simulink model "sm_car_4post_testrig"  (R2021b)
settings: Solver=ode23t  StartTime=0.0  StopTime=20  MaxStep=0.4  RelTol=1e-3  AbsTol=1e-3  EnableMultiTasking=on
PreLoadFcn:
  | sm_car_4post_param
  | sm_car_4post_param_posts
  | load sm_car_4post_op_01
  | load sm_car_4post_op_02
  | load sm_car_4post_op_03
  | 
  | 
  | sm_car_4post_vehicle_01_data
  | sm_car_4post_vehicle_02_data
  | sm_car_4post_vehicle_03_data
  | sm_car_4post_init_data
  | Vehicle = Vehicle_01;
  | sm_car_4post_op = sm_car_4post_op_01;
values from neighbouring files (symbols this model uses):
  brake_pressure_factor = 0.1    [sm_car_4post_param.m]
  brake_rear_factor = 0.3    [sm_car_4post_param.m]
  Init = struct    [sm_car_4post_init_data.m]
  N = 100    [sm_extr_data_cam_roller_curve.m]
  s = sin(q)    [sm_extr_data_cam_roller_curve.m]
  sm_car_4post_op_01 = simscape.op.create(simlog_sm_car_4post,20)    [sm_car_4post_gen_op.m]
  Vehicle_01 = struct    [sm_car_4post_vehicle_01_data.m]
undefined symbols (not defined in the file or in its folder): Axle, Hub, ShaftF, ShaftR, smcar_param, X, xy_data_car_side, xy_data_membrane, Y, Z
libraries: fl_lib x68, sm_lib x50, nesl_utility x40, sm_car_4post_lib x34, simulink x2
(part 1 of 4)
CloseFcn:
  | try,close(h1_sm_car_4post_testrig),end
  | clear h1_sm_car_4post_testrig
  | try,close(h2_sm_car_4post_testrig),end
  | clear h2_sm_car_4post_testrig
  | 
  | clear simlog_sm_car_4post_testrig
  | clear logsout_sm_car_4post_testrig
  | 
  | clear Init
  | clear Vehicle
  | clear Vehicle_01
  | clear Vehicle_02
  | clear Vehicle_03
  | clear brake_pressure_factor
  | clear brake_rear_factor
  | clear sm_car_4post_color
  | clear sm_car_4post_density
  | clear sm_car_4post_op
  | clear sm_car_4post_op_01
  | clear sm_car_4post_op_02
  | clear sm_car_4post_op_03
  | clear sm_car_4post_platform
  | clear smcar_param
  | clear xy_data_membrane
Description:
  | Full Vehicle on Four Post Testrig
settings Model: Creator=The MathWorks, Inc.  LastModifiedBy=The MathWorks, Inc.
settings SolverCC: ConcurrentTasks=on  AlgebraicLoopSolver=TrustRegion  AutoInsertRateTranBlk=on  InsertRTBMode=Never (minimum delay)
settings DataIOCC: MaxDataPoints=10000  SaveFormat=StructureWithTime  ReturnWorkspaceOutputs=off  SignalLoggingName=logsout_sm_car_4post_testrig
settings OptimizationCC: BlockReduction=off  OptimizeBlockIOStorage=off  BufferReuse=off  GlobalBufferReuse=off  ExpressionFolding=off  LocalBlockOutputs=off  OptimizeDataStoreBuffers=off  BusAssignmentInplaceUpdate=off
settings DebuggingCC: SFMachineParentedDataDiag=warning  ArithmeticOperatorsInVariantConditions=warning
settings HardwareCC: ProdBitPerPointer=32  ProdBitPerSizeT=32  ProdBitPerPtrDiffT=32  ProdLargestAtomicFloat=None  ProdWordSize=32  ProdLongLongMode=on  ProdHWDeviceType=Generic->32-bit x86 compatible
settings SFSimCC: CustomCodeUndefinedFunction=UseInterfaceOnly
settings RTWCC: RTWCompilerOptimization=on
settings GRTTargetCC: TargetLangStandard=C89/C90 (ANSI)
settings SimscapeCC: SimscapeLogType=all  SimscapeLogSimulationStatistics=on  SimscapeLogName=simlog_sm_car_4post_testrig  SimscapeLogDataHistory=100000  SimscapeUseOperatingPoints=on  SimscapeOperatingPoint=sm_car_4post_op
settings DiagnosticsConfigSet: SimMechanicsConflictingReferenceFrames=none  SimMechanicsRigidlyBoundBlock=none  SimMechanicsUnsatisfiedHighPriorityTargets=error
settings ExplorerConfigSet: InternalSimMechanicsExplorerSettings="<ExplorerConfiguration><canonicalview>default</canonicalview><AnimationSetting><BasePlaybackSpeed>1.0</BasePlaybackSpeed><PlaybackSpeedFactor>2.0</PlaybackSpeedFactor></AnimationSetting><TilePanel><TileInfo><Tiles Columns=\"2\" Count=\"3\" Rows=\"2\"><Column Weight=\"0.4993\"/><Column Weight=\"0.5007\"/><Row Weight=\"0.5\"/><Row Weight=\"0.5\"/><Tile Height=\"1\" Width=\"1\" X=\"0\" Y=\"0\"/><Tile Height=\"1\" Width=\"1\" X=\"1\" Y=\"0\"/><Tile Height=\"1\" Width=\"2\" X=\"0\" Y=\"1\"/></Tiles></TileInfo><SceneInfo><SceneViewer><BGColor><R>1</R><G>1</G><B>1</B></BGColor><Camera><DoPerspective>off</DoPerspective><Position><X>-193.503182231100908</X><Y>-61.0419033263629984</Y><Z>200.880247292376964</Z></Position><Center><X>-0.0764520266245204833</X><Y>0.688462788949241178</Y><Z>0.441979080031284555</Z></Center><Up><X>0.696897777137974517</X><Y>0.114900599241424928</Y><Z>0.707906307723070949</Z></Up><ViewLimDist>1</ViewLimDist><YLim>0.497951895852590032</YLim><XLim>0.688180709998523321</XLim></Camera></SceneViewer><SceneViewer><BGColor><R>1</R><G>1</G><B>1</B></BGColor><Camera><DoPerspective>off</DoPerspective><Position><X>-1.81478949286671787</X><Y>-285.659072572391551</Y><Z>0.350812117947062074</Z></Position><Center><X>-1.81478949286671787</X><Y>1.0996689468301124e-05</Y><Z>0.350812117947062074</Z></Center><Up><X>0</X><Y>-0</Y><Z>1</Z></Up><ViewLimDist>1</ViewLimDist><YLim>1.90555005908736064</YLim><XLim>2.64064989461544375</XLim></Camera></SceneViewer><SceneViewer><BGColor><R>1</R><G>1</G><B>1</B></BGColor><Camera><DoPerspective>off</DoPerspective><Position><X>174.747144460498959</X><Y>-221.722739064773151</Y><Z>43.636736806567896</Z></Position><Center><X>-1.89730184608775931</X><Y>-0.0435832957411751917</Y><Z>0.499781838173366855</Z></Center><Up><X>-0.0708368498921288503</X><Y>0.13584833277642594</Y><Z>0.988193994709149037</Z></Up><ViewLimDist>1</ViewLimDist><YLim>1.31510781083851214</YLim><XLim>3.68427206931538276</XLim></Camera></SceneViewer></SceneInfo></TilePanel><MechEditorPanel><Cameras><Camera><Id>Camera1</Id><Value><Name>Track Vehicle IsoRF</Name><NativeCamera><PositionTrackingFeature>Camera_Frames.Transform_Camera_BodyIso.F</PositionTrackingFeature><CenterTrackingFeature>Camera_Frames.Transform_Camera_BodyIso_Aim.F</CenterTrackingFeature><UpVectorTrackingFeature>Camera_Frames.Transform_Camera_BodyIso_Aim.F</UpVectorTrackingFeature><CenterTrackingOrigin>off</CenterTrackingOrigin><CenterTrackingDirection>+Y</CenterTrackingDirection><UpVectorTrackingDirection>+Z</UpVectorTrackingDirection></NativeCamera></Value></Camera><Camera><Id>Camera2</Id><Value><Name>Track Vehicle Rear</Name><NativeCamera><PositionTrackingFeature>Camera_Frames.Transform_Camera_Rear.F</PositionTrackingFeature><CenterTrackingFeature>Camera_Frames.Transform_Camera_Rear.F</CenterTrackingFeature><UpVectorTrackingFeature>Camera_Frames.World_Frame.W</UpVectorTrackingFeature><CenterTrackingOrigin>off</CenterTrackingOrigin><CenterTrackingDirection>+X</CenterTrackingDirection><UpVectorTrackingDirection>+Z</UpVectorTrackingDirection></NativeCamera></Value></Camera><Camera><Id>Camera3</Id><Value><Name>Track Vehicle Top</Name><NativeCamera><PositionTrackingFeature>Camera_Frames.Transform_Camera_Top.F</PositionTrackingFeature><CenterTrackingFeature>Camera_Frames.Transform_Camera_Top.F</CenterTrackingFeature><UpVectorTrackingFeature>Camera_Frames.Transform_Camera_Top.F</UpVectorTrackingFeature><CenterTrackingOrigin>off</CenterTrackingOrigin><CenterTrackingDirection>-Z</CenterTrackingDirection><UpVectorTrackingDirection>+X</UpVectorTrackingDirection></NativeCamera></Value></Camera><Camera><Id>Camera4</Id><Value><Name>Track Vehicle Right</Name><NativeCamera><PositionTrackingFeature>Camera_Frames.Transform_Camera_Right.F</PositionTrackingFeature><CenterTrackingFeature>Camera_Frames.Transform_Camera_Right.F</CenterTrackingFeature><UpVectorTrackingFeature>Camera_Frames.World_Frame.W</UpVectorTrackingFeature><CenterTrackingOrigin>off</CenterTrackingOrigin><CenterTrackingDirection>+Y</CenterTrackingDirection><UpVectorTrackingDirection>+Z</UpVectorTrackingDirection></NativeCamera></Value></Camera><Camera><Id>Camera5</Id><Value><Name>Track Susp FR</Name><NativeCamera><PositionTrackingFeature>Camera_Frames.Transform_Camera_Susp_FR.F</PositionTrackingFeature><CenterTrackingFeature>Camera_Frames.Transform_Camera_Susp_FR.F</CenterTrackingFeature><UpVectorTrackingFeature>Camera_Frames.World_Frame.W</UpVectorTrackingFeature><CenterTrackingOrigin>off</CenterTrackingOrigin><CenterTrackingDirection>-X</CenterTrackingDirection><UpVectorTrackingDirection>+Z</UpVectorTrackingDirection></NativeCamera></Value></Camera><Camera><Id>Camera6</Id><Value><Name>Track Susp RR</Name><NativeCamera><PositionTrackingFeature>Camera_Frames.Transform_Camera_Susp_RR.F</PositionTrackingFeature><CenterTrackingFeature>Camera_Frames.Transform_Camera_Susp_RR.F</CenterTrackingFeature><UpVectorTrackingFeature>Camera_Frames.Transform_Camera_Susp_RR.F</UpVectorTrackingFeature><CenterTrackingOrigin>off</CenterTrackingOrigin><CenterTrackingDirection>-X</CenterTrackingDirection><UpVectorTrackingDirection>+Z</UpVectorTrackingDirection></NativeCamera></Value></Camera></Cameras><GfxPanelCameraMap/><VideoCreator><PlaybackSpeedRatio>1.0</PlaybackSpeedRatio><FrameRate>30</FrameRate><VideoFormat>Motion JPEG AVI</VideoFormat><FrameSize>auto</FrameSize></VideoCreator></MechEditorPanel></ExplorerConfiguration>"

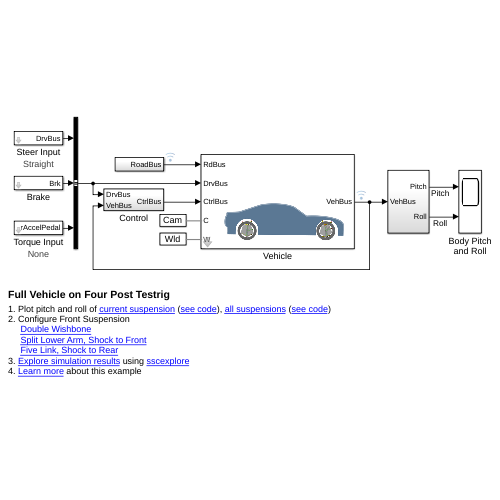
[thumbnail: Simulink's stored preview of the top-level diagram]
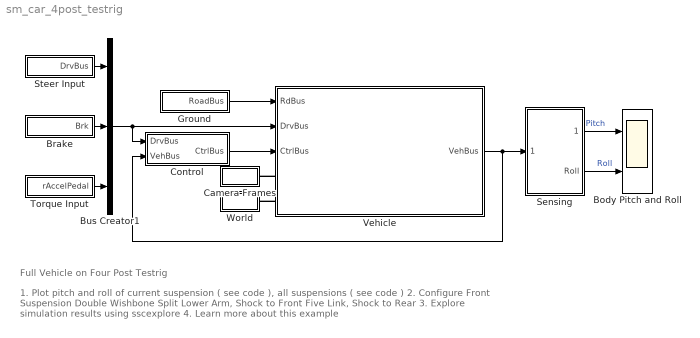
== system sm_car_4post_testrig ==
  note: Full Vehicle on Four Post Testrig
  note: 1. Plot pitch and roll of current suspension ( see code ), all suspensions ( see code )
      | 2. Configure Front Suspension
      | Double Wishbone
      | Split Lower Arm, Shock to Front
      | Five Link, Shock to Rear
      | 3. Explore simulation results using sscexplore
      | 4. Learn more about this example
  Body Pitch and Roll : Scope  NumInputPorts=2
  Brake : Subsystem  mask{brake_on_time=3600}
      mask prompts: brake_on_time "Brake On Time (sec)"
      mask TypeOptions brake_on_time: Step/Time
  Bus Creator1 : BusCreator  Inputs=3
  Camera Frames : Subsystem
      mask Display: disp('Cam')
  Control : Subsystem
  Ground : Subsystem
  Sensing : Subsystem
  Steer Input : Subsystem  mask{popup_steer_input=Straight}
      mask prompts: popup_steer_input "Steer Input"
      settings: AttributesFormatString=%<popup_steer_input>
      mask TypeOptions popup_steer_input: Straight | Step | Sequence | Lane Change
  Torque Input : Subsystem  mask{popup_torque_input=None}
      mask prompts: popup_torque_input "Maneuver Torque"
      mask init:
      | if (popup_torque_input == 1)
      |     rPedalValue = 0.5;
      | elseif (popup_torque_input == 2)
      |     rPedalValue = 0.25;
      | elseif (popup_torque_input == 3)
      |     rPedalValue = 0;
      | end
      settings: AttributesFormatString=%<popup_torque_input>
      mask TypeOptions popup_torque_input: Full Torque | Low Torque | None
  Vehicle : Subsystem  Tag=PublishSubsystem  VariantControl=NS_Con  mask(Vehicle with Multibody Suspension){Vehicle=Vehicle, Init=Init, InitTriggerDropdown=1}
      mask prompts: Vehicle "Vehicle Parameters"; Init "Initial Values"; InitTriggerDropdown "Initialization Trigger Dropdown"
      mask help: Multibody model of a car. All parameter values and the selected suspension configuration are defined by Vehicle Parameters, which must be a specific MATLAB data structure.
      mask init:
      | curblk = gcb;
      | 
      | % Trigger Mask Initialization for 
      | % variant subsystems below this level
      | sm_car_4post_lib_maskInitTrigger(curblk)
      mask TypeOptions InitTriggerDropdown: 0 | 1
      mask DialogControl cont_sim Prompt: Config
      mask Display: image(fullfile(matlabroot,'toolbox','physmod','sm','smdemos','car_4post_testrig','images','sm_car_4post_vehicle_sedan_IMAGE.png'));
  World : Subsystem
      mask Display: disp('Wld')
  wires:
  Bus Creator1/1 -> Control/1(DrvBus), Vehicle/2(DrvBus)
  Steer Input/1(DrvBus) -> Bus Creator1/1
  Brake/1(Brk) -> Bus Creator1/2
  Ground/1(RoadBus) -> Vehicle/1(RdBus)
  Torque Input/1(rAccelPedal) -> Bus Creator1/3
  Control/1(CtrlBus) -> Vehicle/3(CtrlBus)
  Vehicle/1(VehBus) -> Sensing/1(VehBus), Control/2(VehBus)
  Sensing/2(Roll) -> Body Pitch and Roll/2  "Roll"
  Sensing/1(Pitch) -> Body Pitch and Roll/1  "Pitch"
  connections:
  Vehicle/LConn2 -- World/RConn1
  Vehicle/LConn1 -- Camera Frames/RConn1

== system sm_car_4post_testrig/Brake ==
  Step : Step  Time=brake_on_time  After=0.5  SampleTime=0  ZeroCross=off
  Brk : Outport  VectorParamsAs1DForOutWhenUnconnected=off
  wires:
  Step/1 -> Brk/1  "rBrakePedal"

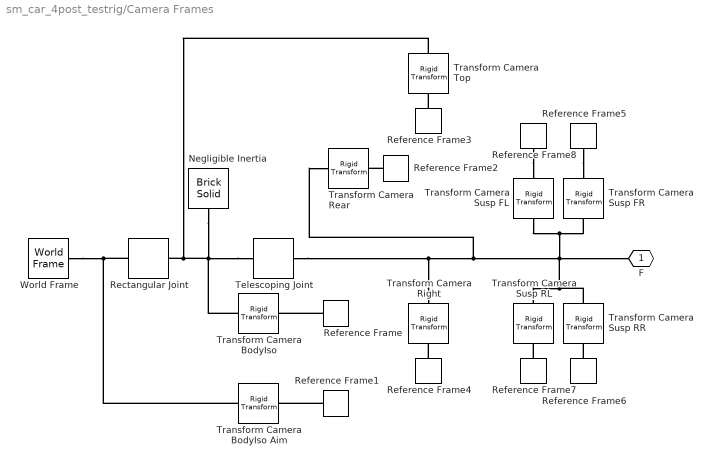
== system sm_car_4post_testrig/Camera Frames ==
  Negligible Inertia : sm_lib/Body Elements/Brick Solid  GraphicAmbientColor=[0.15 0.15 0.15 1.0]  BasedOnType=Density  BrickDimensions=[1 1 1]*1e-3  BrickDimensionUnits=m  CenterOfMass=[0 0 0]  CenterOfMassUnits=m  GraphicDiffuseColor=[0.5 0.5 0.5]  Density=1000  DensityUnits=kg/m^3  DoExposeReferenceFrame=on  GraphicEmissiveColor=[0.0 0.0 0.0 1.0]  ExportEntireGeometry=off  SerializedFrames=<Frames/>  MarkerShape=Sphere  MarkerSize=10  GraphicType=FromGeometry  InertiaType=PointMass  Mass=1e-6  MassUnits=kg  MomentsOfInertia=[1 1 1]  MomentsOfInertiaUnits=kg*m^2  GraphicOpacity=1.0  ProductsOfInertia=[1 1 1]  ProductsOfInertiaUnits=kg*m^2  GraphicShininess=75  GraphicSpecularColor=[0.5 0.5 0.5 1.0]  GraphicVisPropType=SimpleVisualProperties
  Rectangular Joint : sm_lib/Joints/Rectangular Joint  JointMode=Normal  SenseConstraintForce=off  SenseConstraintForceX=off  SenseConstraintForceY=off  SenseConstraintForceZ=off  SenseConstraintTorque=off  SenseConstraintTorqueX=off  SenseConstraintTorqueY=off  SenseConstraintTorqueZ=off  SenseTotalForce=off  SenseTotalForceX=off  SenseTotalForceY=off  SenseTotalForceZ=off  SenseTotalTorque=off  SenseTotalTorqueX=off  SenseTotalTorqueY=off  SenseTotalTorqueZ=off  CompositeWrenchDir=FollowerOnBase  CompositeWrenchFrame=BaseFrame  PxEquilibriumPosition=0  PxEquilibriumPositionUnits=m  PxSpringStiffness=0  PxSpringStiffnessUnits=N/m  PxDampingCoefficient=0  PxDampingCoefficientUnits=N/(m/s)  PxTorqueActuationMode=NoTorque  PxMotionActuationMode=ComputedMotion  PxSensePosition=off  PxSenseVelocity=off  PxSenseAcceleration=off  PxSenseTorqueForce=off  PxSenseLowerLimitTorqueForce=off  PxSenseUpperLimitTorqueForce=off  PxLowerLimitSpecify=off  PxLowerLimitBound=-1  PxLowerLimitBoundUnits=m  PxLowerLimitStiffness=1e6  PxLowerLimitStiffnessUnits=N/m  PxLowerLimitDamping=1e3  PxLowerLimitDampingUnits=N/(m/s)  PxLowerLimitTransitionRegionWidth=1e-4  PxLowerLimitTransitionRegionWidthUnits=m  PxUpperLimitSpecify=off  PxUpperLimitBound=1  PxUpperLimitBoundUnits=m  PxUpperLimitStiffness=1e6  PxUpperLimitStiffnessUnits=N/m  PxUpperLimitDamping=1e3  PxUpperLimitDampingUnits=N/(m/s)  PxUpperLimitTransitionRegionWidth=1e-4  PxUpperLimitTransitionRegionWidthUnits=m  PxPositionTargetSpecify=off  PxPositionTargetPriority=High  PxPositionTargetValue=0  PxPositionTargetValueUnits=m  PxVelocityTargetSpecify=off  PxVelocityTargetPriority=High  PxVelocityTargetValue=0  PxVelocityTargetValueUnits=m/s  PyEquilibriumPosition=0  PyEquilibriumPositionUnits=m  PySpringStiffness=0  PySpringStiffnessUnits=N/m  PyDampingCoefficient=0  PyDampingCoefficientUnits=N/(m/s)  PyTorqueActuationMode=NoTorque  PyMotionActuationMode=ComputedMotion  PySensePosition=off  PySenseVelocity=off  PySenseAcceleration=off  PySenseTorqueForce=off  PySenseLowerLimitTorqueForce=off  PySenseUpperLimitTorqueForce=off  PyLowerLimitSpecify=off  PyLowerLimitBound=-1  PyLowerLimitBoundUnits=m  PyLowerLimitStiffness=1e6  PyLowerLimitStiffnessUnits=N/m  PyLowerLimitDamping=1e3  PyLowerLimitDampingUnits=N/(m/s)  PyLowerLimitTransitionRegionWidth=1e-4  PyLowerLimitTransitionRegionWidthUnits=m  PyUpperLimitSpecify=off  PyUpperLimitBound=1  PyUpperLimitBoundUnits=m  PyUpperLimitStiffness=1e6  PyUpperLimitStiffnessUnits=N/m  PyUpperLimitDamping=1e3  PyUpperLimitDampingUnits=N/(m/s)  PyUpperLimitTransitionRegionWidth=1e-4  PyUpperLimitTransitionRegionWidthUnits=m  PyPositionTargetSpecify=off  PyPositionTargetPriority=High  PyPositionTargetValue=0  PyPositionTargetValueUnits=m  PyVelocityTargetSpecify=off  PyVelocityTargetPriority=High  PyVelocityTargetValue=0  PyVelocityTargetValueUnits=m/s
  Reference Frame{,1..8} (9 alike) : sm_lib/Frames and Transforms/Reference Frame
  Telescoping Joint : sm_lib/Joints/Telescoping Joint  JointMode=Normal  SenseConstraintForce=off  SenseConstraintForceX=off  SenseConstraintForceY=off  SenseConstraintForceZ=off  SenseConstraintTorque=off  SenseConstraintTorqueX=off  SenseConstraintTorqueY=off  SenseConstraintTorqueZ=off  SenseTotalForce=off  SenseTotalForceX=off  SenseTotalForceY=off  SenseTotalForceZ=off  SenseTotalTorque=off  SenseTotalTorqueX=off  SenseTotalTorqueY=off  SenseTotalTorqueZ=off  CompositeWrenchDir=FollowerOnBase  CompositeWrenchFrame=BaseFrame  SphDefPosRotationMethod=None  SphDefPosRotationAngleUnits=deg  SphDefPosRotationStandardAxis=+Z  SphDefPosRotationAngle=0.0  SphDefPosRotationArbitraryAxis=[0 0 1]  SphDefPosFollAlignAxisA=+X  SphDefPosBaseAlignAxisA=+Y  SphDefPosFollAlignAxisB=+Y  SphDefPosBaseAlignAxisB=+Z  SphDefPosRotationSequenceAxes=FollowerAxes  SphDefPosRotationSequence=XYX  SphDefPosRotationSequenceAngles=[0 0 0]  SphDefPosRotationSequenceAnglesUnits=deg  SphDefPosRotationMatrix=[1 0 0; 0 1 0; 0 0 1]  SphEqPosRotationMethod=None  SphEqPosRotationAngleUnits=deg  SphEqPosRotationStandardAxis=+Z  SphEqPosRotationAngle=0.0  SphEqPosRotationArbitraryAxis=[0 0 1]  SphEqPosFollAlignAxisA=+X  SphEqPosBaseAlignAxisA=+Y  SphEqPosFollAlignAxisB=+Y  SphEqPosBaseAlignAxisB=+Z  SphEqPosRotationSequenceAxes=FollowerAxes  SphEqPosRotationSequence=XYX  SphEqPosRotationSequenceAngles=[0 0 0]  SphEqPosRotationSequenceAnglesUnits=deg  SphEqPosRotationMatrix=[1 0 0; 0 1 0; 0 0 1]  SphSpringStiffness=0  SphSpringStiffnessUnits=N*m/deg  SphDampingCoefficient=0  SphDampingCoefficientUnits=N*m/(deg/s)  SphActuateTorqueX=off  SphActuateTorqueY=off  SphActuateTorqueZ=off  SphActuateTorque=off  SphTorqueActuationMode=NoTorque  SphMotionActuationMode=ComputedMotion  SphActuationFrame=BaseFrame  SphSensePosition=off  SphSenseVelocityX=off  SphSenseVelocityY=off  SphSenseVelocityZ=off  SphSenseVelocity=off  SphSenseAccelerationX=off  SphSenseAccelerationY=off  SphSenseAccelerationZ=off  SphSenseAcceleration=off  SphSenseTorqueX=off  SphSenseTorqueY=off  SphSenseTorqueZ=off  SphSenseTorqueForce=off  SphSenseLowerLimitTorqueMag=off  SphSenseUpperLimitTorqueMag=off  SphSensingFrame=BaseFrame  SphLowerLimitSpecify=off  SphLowerLimitBound=15  SphLowerLimitBoundUnits=deg  SphLowerLimitStiffness=1e4  SphLowerLimitStiffnessUnits=N*m/deg  SphLowerLimitDamping=10  SphLowerLimitDampingUnits=N*m/(deg/s)  SphLowerLimitTransitionRegionWidth=0.1  SphLowerLimitTransitionRegionWidthUnits=deg  SphUpperLimitSpecify=off  SphUpperLimitBound=45  SphUpperLimitBoundUnits=deg  SphUpperLimitStiffness=1e4  SphUpperLimitStiffnessUnits=N*m/deg  SphUpperLimitDamping=10  SphUpperLimitDampingUnits=N*m/(deg/s)  SphUpperLimitTransitionRegionWidth=0.1  SphUpperLimitTransitionRegionWidthUnits=deg  SphPositionTargetRotationMethod=None  SphPositionTargetRotationAngleUnits=deg  SphPositionTargetRotationStandardAxis=+Z  SphPositionTargetRotationAngle=0.0  SphPositionTargetRotationArbitraryAxis=[0 0 1]  SphPositionTargetFollAlignAxisA=+X  SphPositionTargetBaseAlignAxisA=+Y  SphPositionTargetFollAlignAxisB=+Y  SphPositionTargetBaseAlignAxisB=+Z  SphPositionTargetRotationSequenceAxes=FollowerAxes  SphPositionTargetRotationSequence=XYX  SphPositionTargetRotationSequenceAngles=[0 0 0]  SphPositionTargetRotationSequenceAnglesUnits=deg  SphPositionTargetRotationMatrix=[1 0 0; 0 1 0; 0 0 1]  SphPositionTargetSpecify=off  SphPositionTargetPriority=High  SphVelocityTargetValue=[0 0 0]  SphVelocityTargetValueUnits=deg/s  SphVelocityTargetSpecify=off  SphVelocityTargetPriority=High  SphVelocityTargetInFollowerFrame=on  PzEquilibriumPosition=0  PzEquilibriumPositionUnits=m  PzSpringStiffness=0  PzSpringStiffnessUnits=N/m  PzDampingCoefficient=0  PzDampingCoefficientUnits=N/(m/s)  PzTorqueActuationMode=NoTorque  PzMotionActuationMode=ComputedMotion  PzSensePosition=off  PzSenseVelocity=off  PzSenseAcceleration=off  PzSenseTorqueForce=off  PzSenseLowerLimitTorqueForce=off  PzSenseUpperLimitTorqueForce=off  PzLowerLimitSpecify=off  PzLowerLimitBound=-1  PzLowerLimitBoundUnits=m  PzLowerLimitStiffness=1e6  PzLowerLimitStiffnessUnits=N/m  PzLowerLimitDamping=1e3  PzLowerLimitDampingUnits=N/(m/s)  PzLowerLimitTransitionRegionWidth=1e-4  PzLowerLimitTransitionRegionWidthUnits=m  PzUpperLimitSpecify=off  PzUpperLimitBound=1  PzUpperLimitBoundUnits=m  PzUpperLimitStiffness=1e6  PzUpperLimitStiffnessUnits=N/m  PzUpperLimitDamping=1e3  PzUpperLimitDampingUnits=N/(m/s)  PzUpperLimitTransitionRegionWidth=1e-4  PzUpperLimitTransitionRegionWidthUnits=m  PzPositionTargetSpecify=off  PzPositionTargetPriority=High  PzPositionTargetValue=0  PzPositionTargetValueUnits=m  PzVelocityTargetSpecify=off  PzVelocityTargetPriority=High  PzVelocityTargetValue=0  PzVelocityTargetValueUnits=m/s
      settings: SourceProductBaseCode=MS
  Transform Camera Rear : sm_lib/Frames and Transforms/Rigid Transform  TranslationMethod=Cartesian  TranslationStandardOffset=0  TranslationLengthUnit=m  TranslationStandardAxis=+Z  TranslationCartesianOffset=[-8-1.6 0 2+0.4225]  TranslationROffset=0  TranslationROffsetUnits=m  TranslationZOffset=0  TranslationZOffsetUnits=m  TranslationThetaOffset=0  TranslationThetaOffsetUnits=deg  RotationMethod=None  RotationAngleUnits=deg  RotationStandardAxis=+Z  RotationAngle=0.0  RotationArbitraryAxis=[0 0 1]  FollAlignAxisA=+X  BaseAlignAxisA=+Y  FollAlignAxisB=+Y  BaseAlignAxisB=+Z  RotationSequenceAxes=FollowerAxes  RotationSequence=XYX  RotationSequenceAngles=[0 0 0]  RotationSequenceAnglesUnits=deg  RotationMatrix=[1 0 0; 0 1 0; 0 0 1]
  Transform Camera Right : sm_lib/Frames and Transforms/Rigid Transform  TranslationMethod=Cartesian  TranslationStandardOffset=0  TranslationLengthUnit=m  TranslationStandardAxis=+Z  TranslationCartesianOffset=[1.5-1.6 -4 0+0.4225]  TranslationROffset=0  TranslationROffsetUnits=m  TranslationZOffset=0  TranslationZOffsetUnits=m  TranslationThetaOffset=0  TranslationThetaOffsetUnits=deg  RotationMethod=None  RotationAngleUnits=deg  RotationStandardAxis=+Z  RotationAngle=0.0  RotationArbitraryAxis=[0 0 1]  FollAlignAxisA=+X  BaseAlignAxisA=+Y  FollAlignAxisB=+Y  BaseAlignAxisB=+Z  RotationSequenceAxes=FollowerAxes  RotationSequence=XYX  RotationSequenceAngles=[0 0 0]  RotationSequenceAnglesUnits=deg  RotationMatrix=[1 0 0; 0 1 0; 0 0 1]
  Transform Camera Susp FL : sm_lib/Frames and Transforms/Rigid Transform  TranslationMethod=Cartesian  TranslationStandardOffset=0  TranslationLengthUnit=m  TranslationStandardAxis=+Z  TranslationCartesianOffset=[-0.9 0.45 0.35]  TranslationROffset=0  TranslationROffsetUnits=m  TranslationZOffset=0  TranslationZOffsetUnits=m  TranslationThetaOffset=0  TranslationThetaOffsetUnits=deg  RotationMethod=StandardAxis  RotationAngleUnits=deg  RotationStandardAxis=+Z  RotationAngle=180  RotationArbitraryAxis=[0 0 1]  FollAlignAxisA=+X  BaseAlignAxisA=+Y  FollAlignAxisB=+Y  BaseAlignAxisB=+Z  RotationSequenceAxes=FollowerAxes  RotationSequence=XYX  RotationSequenceAngles=[0 0 0]  RotationSequenceAnglesUnits=deg  RotationMatrix=[1 0 0; 0 1 0; 0 0 1]
  Transform Camera Susp FR : sm_lib/Frames and Transforms/Rigid Transform  TranslationMethod=Cartesian  TranslationStandardOffset=0  TranslationLengthUnit=m  TranslationStandardAxis=+Z  TranslationCartesianOffset=[-0.9 -0.45 0.35]  TranslationROffset=0  TranslationROffsetUnits=m  TranslationZOffset=0  TranslationZOffsetUnits=m  TranslationThetaOffset=0  TranslationThetaOffsetUnits=deg  RotationMethod=StandardAxis  RotationAngleUnits=deg  RotationStandardAxis=+Z  RotationAngle=180  RotationArbitraryAxis=[0 0 1]  FollAlignAxisA=+X  BaseAlignAxisA=+Y  FollAlignAxisB=+Y  BaseAlignAxisB=+Z  RotationSequenceAxes=FollowerAxes  RotationSequence=XYX  RotationSequenceAngles=[0 0 0]  RotationSequenceAnglesUnits=deg  RotationMatrix=[1 0 0; 0 1 0; 0 0 1]
  Transform Camera Susp RL : sm_lib/Frames and Transforms/Rigid Transform  TranslationMethod=Cartesian  TranslationStandardOffset=0  TranslationLengthUnit=m  TranslationStandardAxis=+Z  TranslationCartesianOffset=[-2.6 0.45 0.35]  TranslationROffset=0  TranslationROffsetUnits=m  TranslationZOffset=0  TranslationZOffsetUnits=m  TranslationThetaOffset=0  TranslationThetaOffsetUnits=deg  RotationMethod=StandardAxis  RotationAngleUnits=deg  RotationStandardAxis=+Z  RotationAngle=0  RotationArbitraryAxis=[0 0 1]  FollAlignAxisA=+X  BaseAlignAxisA=+Y  FollAlignAxisB=+Y  BaseAlignAxisB=+Z  RotationSequenceAxes=FollowerAxes  RotationSequence=XYX  RotationSequenceAngles=[0 0 0]  RotationSequenceAnglesUnits=deg  RotationMatrix=[1 0 0; 0 1 0; 0 0 1]
  Transform Camera Susp RR : sm_lib/Frames and Transforms/Rigid Transform  TranslationMethod=Cartesian  TranslationStandardOffset=0  TranslationLengthUnit=m  TranslationStandardAxis=+Z  TranslationCartesianOffset=[-2.6 -0.45 0.35]  TranslationROffset=0  TranslationROffsetUnits=m  TranslationZOffset=0  TranslationZOffsetUnits=m  TranslationThetaOffset=0  TranslationThetaOffsetUnits=deg  RotationMethod=StandardAxis  RotationAngleUnits=deg  RotationStandardAxis=+Z  RotationAngle=0  RotationArbitraryAxis=[0 0 1]  FollAlignAxisA=+X  BaseAlignAxisA=+Y  FollAlignAxisB=+Y  BaseAlignAxisB=+Z  RotationSequenceAxes=FollowerAxes  RotationSequence=XYX  RotationSequenceAngles=[0 0 0]  RotationSequenceAnglesUnits=deg  RotationMatrix=[1 0 0; 0 1 0; 0 0 1]
  Transform Camera Top : sm_lib/Frames and Transforms/Rigid Transform  TranslationMethod=Cartesian  TranslationStandardOffset=0  TranslationLengthUnit=m  TranslationStandardAxis=+Z  TranslationCartesianOffset=[-1.6 0 12+0.4225]  TranslationROffset=0  TranslationROffsetUnits=m  TranslationZOffset=0  TranslationZOffsetUnits=m  TranslationThetaOffset=0  TranslationThetaOffsetUnits=deg  RotationMethod=None  RotationAngleUnits=deg  RotationStandardAxis=+Z  RotationAngle=0.0  RotationArbitraryAxis=[0 0 1]  FollAlignAxisA=+X  BaseAlignAxisA=+Y  FollAlignAxisB=+Y  BaseAlignAxisB=+Z  RotationSequenceAxes=FollowerAxes  RotationSequence=XYX  RotationSequenceAngles=[0 0 0]  RotationSequenceAnglesUnits=deg  RotationMatrix=[1 0 0; 0 1 0; 0 0 1]
  Transform Camera BodyIso : sm_lib/Frames and Transforms/Rigid Transform  TranslationMethod=Cartesian  TranslationStandardOffset=0  TranslationLengthUnit=m  TranslationStandardAxis=+Z  TranslationCartesianOffset=[2.5-1.6 -5.0 1+0.4225]  TranslationROffset=0  TranslationROffsetUnits=m  TranslationZOffset=0  TranslationZOffsetUnits=m  TranslationThetaOffset=0  TranslationThetaOffsetUnits=deg  RotationMethod=None  RotationAngleUnits=deg  RotationStandardAxis=+Z  RotationAngle=0.0  RotationArbitraryAxis=[0 0 1]  FollAlignAxisA=+X  BaseAlignAxisA=+Y  FollAlignAxisB=+Y  BaseAlignAxisB=+Z  RotationSequenceAxes=FollowerAxes  RotationSequence=XYX  RotationSequenceAngles=[0 0 0]  RotationSequenceAnglesUnits=deg  RotationMatrix=[1 0 0; 0 1 0; 0 0 1]
  Transform Camera BodyIso Aim : sm_lib/Frames and Transforms/Rigid Transform  TranslationMethod=StandardAxis  TranslationStandardOffset=1.6  TranslationLengthUnit=m  TranslationStandardAxis=+X  TranslationCartesianOffset=[0 0 0]  TranslationROffset=0  TranslationROffsetUnits=m  TranslationZOffset=0  TranslationZOffsetUnits=m  TranslationThetaOffset=0  TranslationThetaOffsetUnits=deg  RotationMethod=RotationSequence  RotationAngleUnits=deg  RotationStandardAxis=+Y  RotationAngle=60  RotationArbitraryAxis=[0 0 1]  FollAlignAxisA=+X  BaseAlignAxisA=+Y  FollAlignAxisB=+Y  BaseAlignAxisB=+Z  RotationSequenceAxes=FollowerAxes  RotationSequence=ZXZ  RotationSequenceAngles=[25 -10 0+0.4225]  RotationSequenceAnglesUnits=deg  RotationMatrix=[1 0 0; 0 1 0; 0 0 1]
  World Frame : sm_lib/Frames and Transforms/World Frame
  F : PMIOPort  Side=Right
  connections:
  Reference Frame8/RConn1 -- Transform Camera Susp FL/RConn1
  Reference Frame7/RConn1 -- Transform Camera Susp RL/RConn1
  Reference Frame6/RConn1 -- Transform Camera Susp RR/RConn1
  Reference Frame5/RConn1 -- Transform Camera Susp FR/RConn1
  Reference Frame4/RConn1 -- Transform Camera Right/RConn1
  Reference Frame3/RConn1 -- Transform Camera Top/RConn1
  Reference Frame2/RConn1 -- Transform Camera Rear/RConn1
  Reference Frame1/RConn1 -- Transform Camera BodyIso Aim/RConn1
  Reference Frame/RConn1 -- Transform Camera BodyIso/RConn1
  Telescoping Joint/RConn1 -- Negligible Inertia/RConn1 -- Rectangular Joint/RConn1 -- Transform Camera Top/LConn1 -- Transform Camera BodyIso/LConn1
  Transform Camera Right/LConn1 -- Transform Camera Rear/LConn1 -- Transform Camera Susp FL/LConn1 -- Transform Camera Susp FR/LConn1 -- F/RConn1 -- Transform Camera Susp RL/LConn1 -- Transform Camera Susp RR/LConn1 -- Telescoping Joint/LConn1
  World Frame/RConn1 -- Transform Camera BodyIso Aim/LConn1 -- Rectangular Joint/LConn1

== system sm_car_4post_testrig/Control ==
  In Bus Element1 : Inport  PortName=DrvBus  Element=rAccelPedal
  In Bus Element2 : Inport  PortName=DrvBus  Element=rBrakePedal
  VehBus : Inport  Port=2
  Bus Creator1 : BusCreator  Inputs=4
  Bus Creator2 : BusCreator  Inputs=4
  Driveline Control : Subsystem
  Pedal : Subsystem  VariantControl=Pedal
  Power Control : Subsystem
  Spring Damper : Subsystem
  Susp : Subsystem
  CtrlBus : Outport  VectorParamsAs1DForOutWhenUnconnected=off
  wires:
  Driveline Control/1(Driveline) -> Bus Creator2/3
  Bus Creator2/1 -> CtrlBus/1
  Bus Creator1/1 -> Bus Creator2/1  "Chassis"
  VehBus/1 -> Pedal/2(VehBus), Power Control/2(VehBus)
  Pedal/1(Brakes) -> Bus Creator2/4
  Power Control/1(Power) -> Bus Creator2/2
  In Bus Element2/1 -> Pedal/1(rBrakePedal)
  In Bus Element1/1 -> Power Control/1(rAccelPedal)
  Susp/1(SuspF) -> Bus Creator1/1
  Spring Damper/2(Spring) -> Bus Creator1/4
  Spring Damper/1(Damper) -> Bus Creator1/3
  Susp/2(SuspR) -> Bus Creator1/2

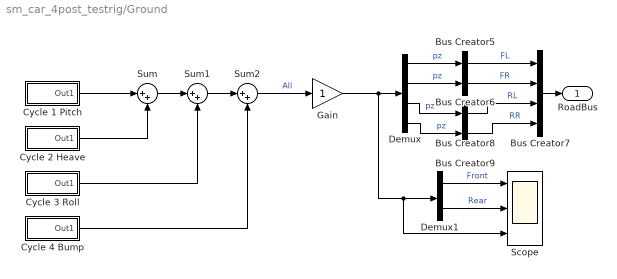
== system sm_car_4post_testrig/Ground ==
  Bus Creator{5..6,8..9} (4 alike) : BusCreator  Inputs=1
  Bus Creator7 : BusCreator  Inputs=4
  Cycle 1 Pitch : Subsystem
  Cycle 2 Heave : Subsystem
  Cycle 3 Roll : Subsystem
  Cycle 4 Bump : Subsystem
  Demux : Demux
  Demux1 : Demux  Outputs=2
  Gain : Gain
  Scope : Scope  NumInputPorts=3
  Sum : Sum  Inputs=|++
  Sum1 : Sum  Inputs=|++
  Sum2 : Sum  Inputs=|++
  RoadBus : Outport  VectorParamsAs1DForOutWhenUnconnected=off
  wires:
  Cycle 2 Heave/1(Out1) -> Sum/2
  Sum2/1 -> Gain/1  "All"
  Demux/1 -> Bus Creator5/1  "pz"
  Demux/2 -> Bus Creator6/1  "pz"
  Bus Creator5/1 -> Bus Creator7/1  "FL"
  Bus Creator6/1 -> Bus Creator7/2  "FR"
  Bus Creator9/1 -> Bus Creator7/4  "RR"
  Bus Creator8/1 -> Bus Creator7/3  "RL"
  Demux/4 -> Bus Creator9/1  "pz"
  Demux/3 -> Bus Creator8/1  "pz"
  Bus Creator7/1 -> RoadBus/1
  Cycle 1 Pitch/1(Out1) -> Sum/1
  Sum/1 -> Sum1/1
  Cycle 3 Roll/1(Out1) -> Sum1/2
  Sum1/1 -> Sum2/1
  Cycle 4 Bump/1(Out1) -> Sum2/2
  Demux1/1 -> Scope/1  "Front"
  Demux1/2 -> Scope/2  "Rear"
  Gain/1 -> Scope/3, Demux1/1, Demux/1

== system sm_car_4post_testrig/Sensing ==
  VehBus : Inport
  Bus Selector1 : BusSelector  OutputSignals=Body.aPitch,Body.aRoll
  Gain : Gain  Gain=180/pi
  Gain1 : Gain  Gain=180/pi
  Pitch : Outport  VectorParamsAs1DForOutWhenUnconnected=off
  Roll : Outport  Port=2  VectorParamsAs1DForOutWhenUnconnected=off
  wires:
  VehBus/1 -> Bus Selector1/1
  Bus Selector1/2 -> Gain/1  "<aRoll>"
  Bus Selector1/1 -> Gain1/1  "<aPitch>"
  Gain/1 -> Roll/1
  Gain1/1 -> Pitch/1

== system sm_car_4post_testrig/Steer Input ==
  Constant : Constant  Value=popup_steer_input
  Lane Change : simulink/Sources/Repeating Sequence  rep_seq_t=[0 10 10.5 11.5 12 13 13.5 20]  rep_seq_y=[0 0 1 1 -1 -1 0 0]*5
  Multiport Switch : MultiPortSwitch  Inputs=4
  No Steer : Constant  Value=0
  Sequence : simulink/Sources/Repeating Sequence  rep_seq_t=[0 1 2 3 4 5]  rep_seq_y=[0 0 -1 1 0 0]*5
  Step : Step  Time=5  After=5  SampleTime=0  ZeroCross=off
      settings: AttributesFormatString=%<After> @ %<Time> sec
  DrvBus : Outport  VectorParamsAs1DForOutWhenUnconnected=off
  wires:
  Lane Change/1 -> Multiport Switch/5  "aStrWhlF"
  Multiport Switch/1 -> DrvBus/1  "aSteerWheel"
  No Steer/1 -> Multiport Switch/2
  Step/1 -> Multiport Switch/3  "aStrWhlF"
  Constant/1 -> Multiport Switch/1
  Sequence/1 -> Multiport Switch/4  "aStrWhlF"

== system sm_car_4post_testrig/Torque Input ==
  Torque Front : Subsystem  mask{on_time=1, off_time=2, rPedalValue=rPedalValue}
      mask prompts: on_time "On Time (s)"; off_time "Off Time (s)"; rPedalValue "Torque Value (N*m)"
      mask TypeOptions on_time: Step On/Time
      mask TypeOptions off_time: Step Off/Time
      mask TypeOptions rPedalValue: Gain/Gain
  rAccelPedal : Outport  VectorParamsAs1DForOutWhenUnconnected=off
  wires:
  Torque Front/1(rAccelPedal) -> rAccelPedal/1  "rAccelPedal"

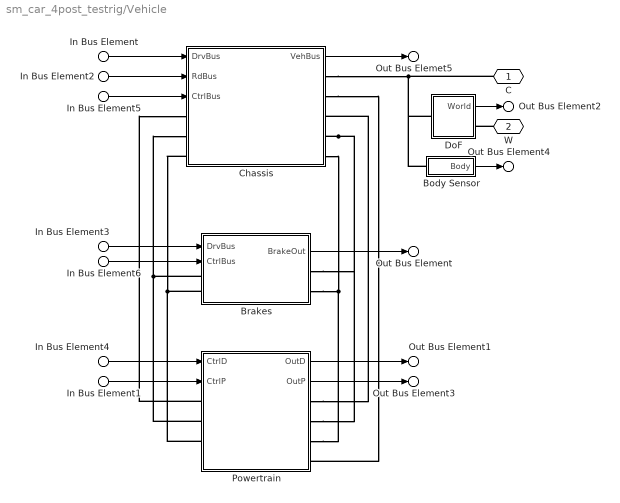
== system sm_car_4post_testrig/Vehicle ==
  In Bus Element2 : Inport  PortName=RdBus
  In Bus Element : Inport  Port=2  PortName=DrvBus
  In Bus Element3 : Inport  Port=2  PortName=DrvBus
  In Bus Element6 : Inport  Port=3  PortName=CtrlBus  Element=Brakes
  In Bus Element5 : Inport  Port=3  PortName=CtrlBus  Element=Chassis
  In Bus Element1 : Inport  Port=3  PortName=CtrlBus  Element=Power
  In Bus Element4 : Inport  Port=3  PortName=CtrlBus  Element=Driveline
  Body Sensor : Subsystem
  Brakes : Subsystem  mask(Brakes){Brakes=Vehicle.Brakes}
      mask prompts: Brakes "Brake Parameters"
      mask help: Brakes for each wheel in a four-wheeled vehicle.
      mask Display: image(fullfile(matlabroot,'toolbox','physmod','sm','smdemos','car_4post_testrig','images','sm_car_4post_variant_brakes_IMAGE.png'));
  Chassis : Subsystem  Tag=PublishSubsystem  VariantControl=Chassis  mask(Vehicle Chassis){Chassis=Vehicle.Chassis, Init=Init, InitTriggerDropdown=1}
      mask prompts: Chassis "Vehicle Parameters"; Init "Initial Values"; InitTriggerDropdown "Initialization Trigger Dropdown"
      mask help: Multibody model of vehicle chassis, including suspension and wheels.
      mask init:
      | curblk = gcb;
      | 
      | % Trigger Mask Initialization for 
      | % variant subsystems below this level
      | sm_car_4post_lib_maskInitTrigger(curblk)
      mask TypeOptions InitTriggerDropdown: 0 | 1
      mask Display: image(fullfile(matlabroot,'toolbox','physmod','sm','smdemos','car_4post_testrig','images','sm_car_4post_variant_chassis_IMAGE.png'));
  DoF : Subsystem  mask(Sensor, World Frame){Init=Init.Chassis}
      mask prompts: Init "Initial Values"
      mask help: Specifies initial vehicle position and speed. Takes vehicle measurements in World Frame.
  Powertrain : Subsystem  mask(Powertrain){Powertrain=Vehicle.Powertrain, InitTriggerDropdown=1}
      mask prompts: Powertrain "Powertrain Parameters"; InitTriggerDropdown "Initialization Trigger Dropdown"
      mask help: Powertrain subsystem for vehicle.
      mask init:
      | curblk = gcb;
      | 
      | % Trigger Mask Initialization for 
      | % variant subsystems below this level
      | sm_car_4post_lib_maskInitTrigger(curblk)
      mask TypeOptions InitTriggerDropdown: 0 | 1
      mask Display: image(fullfile(matlabroot,'toolbox','physmod','sm','smdemos','car_4post_testrig','images','sm_car_4post_variant_powertrain_IMAGE.png'));
  C : PMIOPort  Side=Left
  W : PMIOPort  Port=2  Side=Left
  Out Bus Element4 : Outport  VectorParamsAs1DForOutWhenUnconnected=off  PortName=VehBus  Element=Body
  Out Bus Elemet5 : Outport  VectorParamsAs1DForOutWhenUnconnected=off  PortName=VehBus  Element=Chassis
  Out Bus Element : Outport  VectorParamsAs1DForOutWhenUnconnected=off  PortName=VehBus  Element=Brakes
  Out Bus Element1 : Outport  VectorParamsAs1DForOutWhenUnconnected=off  PortName=VehBus  Element=Driveline
  Out Bus Element2 : Outport  VectorParamsAs1DForOutWhenUnconnected=off  PortName=VehBus  Element=World
  Out Bus Element3 : Outport  VectorParamsAs1DForOutWhenUnconnected=off  PortName=VehBus  Element=Power
  wires:
  Powertrain/2(OutP) -> Out Bus Element3/1
  Powertrain/1(OutD) -> Out Bus Element1/1
  In Bus Element1/1 -> Powertrain/2(CtrlP)
  In Bus Element4/1 -> Powertrain/1(CtrlD)
  In Bus Element3/1 -> Brakes/1(DrvBus)
  DoF/1(World) -> Out Bus Element2/1
  Body Sensor/1(Body) -> Out Bus Element4/1
  In Bus Element6/1 -> Brakes/2(CtrlBus)
  In Bus Element/1 -> Chassis/1(DrvBus)
  In Bus Element2/1 -> Chassis/2(RdBus)
  Chassis/1(VehBus) -> Out Bus Elemet5/1
  Brakes/1(BrakeOut) -> Out Bus Element/1
  In Bus Element5/1 -> Chassis/3(CtrlBus)
  connections:
  Powertrain/RConn1 -- Chassis/RConn3
  Powertrain/LConn1 -- Chassis/LConn1
  Chassis/RConn2 -- Powertrain/RConn4
  Powertrain/LConn2 -- Brakes/LConn1 -- Chassis/LConn2
  Chassis/RConn4 -- Brakes/RConn1 -- Powertrain/RConn2
  Powertrain/RConn3 -- Brakes/RConn2 -- Chassis/RConn5
  Powertrain/LConn3 -- Brakes/LConn2 -- Chassis/LConn3
  W/RConn1 -- DoF/RConn1
  Chassis/RConn1 -- Body Sensor/LConn1 -- DoF/LConn1 -- C/RConn1

== system sm_car_4post_testrig/World ==
  MechanismConfiguration : sm_lib/Utilities/Mechanism Configuration  UniformGravity=Constant  GravityVector=[0 0 -9.80665]  GravityUnits=m/s^2  LinearizationDelta=0.001  JointModeTransitionNonlinearIterations=2
  Solver Configuration : nesl_utility/Solver Configuration  PhysicalDomain=network_engine_domain  SubClassName=solver  LeftPortType=input  RightPortType=generic  Tones=[]  Harmonics=[]  SimulateNoise=off  Profile=off  UseLocalSampling=off  EnableSwitchedLinearOptims=on  FrequencyDomain=off  UseCCode=off  RelTol=0.001  AbsTol=1e-06  MinStep=1e-09  ToWorkspace=off  RevertToSquareIcSolve=off  NumHomotopyIterations=100  PhasorMode=off  PhasorModeNumHarmonics=1  DoDC=off  ResidualTolerance=1e-9  UseLocalSolver=off  LocalSolverChoice=NE_BACKWARD_EULER_ADVANCER  LocalSolverSampleTime=0.005  DoFixedCost=off  MaxNonlinIter=3  MaxModeIter=2  ComputeImpulses=off  ImpulseIterations=2  LinearAlgebra=Sparse  EquationFormulation=NE_TIME_EF  DelaysMemoryBudget=1024  AutomaticFiltering=on  FilteringTimeConstant=0.001  PartitionStorageMethod=AS_NEEDED  PartitionMemoryBudget=1024  PartitionMethod=FAST
      settings: SourceProductBaseCode=PW,SS
  World Frame : sm_lib/Frames and Transforms/World Frame
  W : PMIOPort  Side=Right
  connections:
  Solver Configuration/RConn1 -- World Frame/RConn1 -- W/RConn1 -- MechanismConfiguration/RConn1

== system sm_car_4post_testrig/Control/Driveline Control ==
  Bus Creator : BusCreator  Inputs=1
  Constant : Constant  Value=0
  Driveline : Outport  VectorParamsAs1DForOutWhenUnconnected=off
  wires:
  Constant/1 -> Bus Creator/1  "placeholder"
  Bus Creator/1 -> Driveline/1  "Driveline"

== system sm_car_4post_testrig/Control/Pedal ==
  rBrakePedal : Inport
  VehBus : Inport  Port=2
  Apply{,1..3} (4 alike) : Constant  Value=[0 1]
  Bus Creator : BusCreator  Inputs=1
  Bus Creator1 : BusCreator  Inputs=4
  Terminator : Terminator
  Terminator1 : Terminator
  Brakes : Outport  VectorParamsAs1DForOutWhenUnconnected=off
  wires:
  rBrakePedal/1 -> Terminator1/1
  Apply3/1 -> Bus Creator1/4  "RR"
  Apply2/1 -> Bus Creator1/3  "RL"
  Apply1/1 -> Bus Creator1/2  "FR"
  Apply/1 -> Bus Creator1/1  "FL"
  Bus Creator1/1 -> Bus Creator/1  "Valves"
  VehBus/1 -> Terminator/1
  Bus Creator/1 -> Brakes/1  "Brakes"

== system sm_car_4post_testrig/Control/Power Control ==
  rAccelPedal : Inport
  VehBus : Inport  Port=2
  Bus Creator : BusCreator  Inputs=3
  Constant : Constant  Value=0
  Constant1 : Constant  Value=0
  Gain : Gain  Gain=1600
  Rate Limiter : RateLimiter  RisingSlewLimit=300  FallingSlewLimit=-5000  SampleTimeMode=inherited
  Terminator : Terminator
  Power : Outport  VectorParamsAs1DForOutWhenUnconnected=off
  wires:
  Constant1/1 -> Bus Creator/3  "MRegenBrakeLimit"
  VehBus/1 -> Terminator/1
  rAccelPedal/1 -> Gain/1
  Constant/1 -> Bus Creator/1  "MMotorFDemand"
  Gain/1 -> Rate Limiter/1
  Rate Limiter/1 -> Bus Creator/2  "MMotorRDemand"
  Bus Creator/1 -> Power/1  "Power"

== system sm_car_4post_testrig/Control/Spring Damper ==
  Bus Creator : BusCreator  Inputs=4
  Bus Creator1 : BusCreator  Inputs=4
  Constant : Constant  Value=[0 0 0 0]
  Constant1 : Constant  Value=[0 0 0 0]
  Demux : Demux
  Demux1 : Demux
  Damper : Outport  VectorParamsAs1DForOutWhenUnconnected=off
  Spring : Outport  Port=2  VectorParamsAs1DForOutWhenUnconnected=off
  wires:
  Bus Creator/1 -> Spring/1  "Spring"
  Bus Creator1/1 -> Damper/1  "Damper"
  Constant1/1 -> Demux1/1
  Demux1/3 -> Bus Creator1/3  "RL"
  Demux1/4 -> Bus Creator1/4  "RR"
  Demux1/1 -> Bus Creator1/1  "FL"
  Demux1/2 -> Bus Creator1/2  "FR"
  Demux/2 -> Bus Creator/2  "FR"
  Demux/1 -> Bus Creator/1  "FL"
  Demux/4 -> Bus Creator/4  "RR"
  Demux/3 -> Bus Creator/3  "RL"
  Constant/1 -> Demux/1

== system sm_car_4post_testrig/Control/Susp ==
  Bus Creator1 : BusCreator  Inputs=1
  Bus Creator2 : BusCreator  Inputs=1
  Bus Creator3 : BusCreator  Inputs=1
  Constant1 : Constant  Value=0
  Steer : Subsystem
  SuspF : Outport  VectorParamsAs1DForOutWhenUnconnected=off
  SuspR : Outport  Port=2  VectorParamsAs1DForOutWhenUnconnected=off
  wires:
  Steer/1(Steer) -> Bus Creator1/1
  Constant1/1 -> Bus Creator2/1  "iMotor"
  Bus Creator2/1 -> Bus Creator3/1  "Steer"
  Bus Creator3/1 -> SuspR/1  "SuspR"
  Bus Creator1/1 -> SuspF/1  "SuspF"

== system sm_car_4post_testrig/Ground/Cycle 1 Pitch ==
  Mux : Mux  Inputs=2
  Mux1 : Mux  Inputs=2
  Mux3 : Mux  Inputs=2
  Sine Input FL : sm_car_4post_lib/Sine Input  wave_period=2  num_periods=2  wave_amplitude=0.05  wave_delay=1
      settings: SourceProductBaseCode=MS
  Sine Input FR : sm_car_4post_lib/Sine Input  wave_period=2  num_periods=2  wave_amplitude=0.05  wave_delay=1
      settings: SourceProductBaseCode=MS
  Sine Input RL : sm_car_4post_lib/Sine Input  wave_period=2  num_periods=2  wave_amplitude=0.05  wave_delay=1.5
      settings: SourceProductBaseCode=MS
  Sine Input RR : sm_car_4post_lib/Sine Input  wave_period=2  num_periods=2  wave_amplitude=0.05  wave_delay=1.5
      settings: SourceProductBaseCode=MS
  Out1 : Outport  VectorParamsAs1DForOutWhenUnconnected=off
  wires:
  Sine Input FL/1 -> Mux/1
  Sine Input FR/1 -> Mux/2
  Mux/1 -> Mux3/1
  Mux3/1 -> Out1/1
  Mux1/1 -> Mux3/2
  Sine Input RR/1 -> Mux1/2
  Sine Input RL/1 -> Mux1/1

== system sm_car_4post_testrig/Ground/Cycle 2 Heave ==
  Mux : Mux  Inputs=2
  Mux1 : Mux  Inputs=2
  Mux3 : Mux  Inputs=2
  Sine Input FL : sm_car_4post_lib/Sine Input  wave_period=2  num_periods=2  wave_amplitude=0.05  wave_delay=6
      settings: SourceProductBaseCode=MS
  Sine Input FR : sm_car_4post_lib/Sine Input  wave_period=2  num_periods=2  wave_amplitude=0.05  wave_delay=6
      settings: SourceProductBaseCode=MS
  Sine Input RL : sm_car_4post_lib/Sine Input  wave_period=2  num_periods=2  wave_amplitude=0.05  wave_delay=6
      settings: SourceProductBaseCode=MS
  Sine Input RR : sm_car_4post_lib/Sine Input  wave_period=2  num_periods=2  wave_amplitude=0.05  wave_delay=6
      settings: SourceProductBaseCode=MS
  Out1 : Outport  VectorParamsAs1DForOutWhenUnconnected=off
  wires:
  Sine Input RL/1 -> Mux1/1
  Sine Input RR/1 -> Mux1/2
  Mux1/1 -> Mux3/2
  Mux3/1 -> Out1/1
  Mux/1 -> Mux3/1
  Sine Input FR/1 -> Mux/2
  Sine Input FL/1 -> Mux/1

== system sm_car_4post_testrig/Ground/Cycle 3 Roll ==
  Mux : Mux  Inputs=2
  Mux1 : Mux  Inputs=2
  Mux3 : Mux  Inputs=2
  Sine Input FL : sm_car_4post_lib/Sine Input  wave_period=1  num_periods=3  wave_amplitude=0.03  wave_delay=11
      settings: SourceProductBaseCode=MS
  Sine Input FR : sm_car_4post_lib/Sine Input  wave_period=1  num_periods=3  wave_amplitude=0.03  wave_delay=11.5
      settings: SourceProductBaseCode=MS
  Sine Input RL : sm_car_4post_lib/Sine Input  wave_period=1  num_periods=3  wave_amplitude=0.03  wave_delay=11
      settings: SourceProductBaseCode=MS
  Sine Input RR : sm_car_4post_lib/Sine Input  wave_period=1  num_periods=3  wave_amplitude=0.03  wave_delay=11.5
      settings: SourceProductBaseCode=MS
  Out1 : Outport  VectorParamsAs1DForOutWhenUnconnected=off
  wires:
  Sine Input FL/1 -> Mux/1
  Sine Input FR/1 -> Mux/2
  Mux/1 -> Mux3/1
  Mux3/1 -> Out1/1
  Mux1/1 -> Mux3/2
  Sine Input RR/1 -> Mux1/2
  Sine Input RL/1 -> Mux1/1

== system sm_car_4post_testrig/Ground/Cycle 4 Bump ==
  Mux : Mux  Inputs=2
  Mux2 : Mux  Inputs=2
  Mux3 : Mux  Inputs=2
  Pulse Input : sm_car_4post_lib/Pulse Input  rise_time=0.1  pulse_length=2  wave_amplitude=0.05  wave_delay=15
      settings: SourceProductBaseCode=MS
  Pulse Input1 : sm_car_4post_lib/Pulse Input  rise_time=0.1  pulse_length=2  wave_amplitude=0.05  wave_delay=15
      settings: SourceProductBaseCode=MS
  Pulse Input2 : sm_car_4post_lib/Pulse Input  rise_time=0.1  pulse_length=2  wave_amplitude=0.05  wave_delay=15.5
      settings: SourceProductBaseCode=MS
  Pulse Input3 : sm_car_4post_lib/Pulse Input  rise_time=0.1  pulse_length=2  wave_amplitude=0.05  wave_delay=15.5
      settings: SourceProductBaseCode=MS
  Out1 : Outport  VectorParamsAs1DForOutWhenUnconnected=off
  wires:
  Mux2/1 -> Mux3/2
  Mux3/1 -> Out1/1
  Mux/1 -> Mux3/1
  Pulse Input3/1 -> Mux2/2
  Pulse Input1/1 -> Mux/2
  Pulse Input/1 -> Mux/1
  Pulse Input2/1 -> Mux2/1

== system sm_car_4post_testrig/Torque Input/Torque Front ==
  Gain : Gain  Gain=rPedalValue
  Step Off : Step  Time=off_time  After=-1  SampleTime=0  ZeroCross=off
  Step On : Step  Time=on_time  SampleTime=0  ZeroCross=off
  Sum : Sum  Inputs=|++
  rAccelPedal : Outport  VectorParamsAs1DForOutWhenUnconnected=off
  wires:
  Gain/1 -> rAccelPedal/1  "rAccelPedal"
  Step On/1 -> Sum/1
  Step Off/1 -> Sum/2
  Sum/1 -> Gain/1
